simulink model "lab1_1"  (R2020b)
settings: Solver=VariableStepAuto  StartTime=0.0  StopTime=50  MaxStep=0.01  RelTol=1e-3
InitFcn:
  | lambda = 5;
  | theta = 5;
settings Model: Creator=Eeer12  LastModifiedBy=Eugene

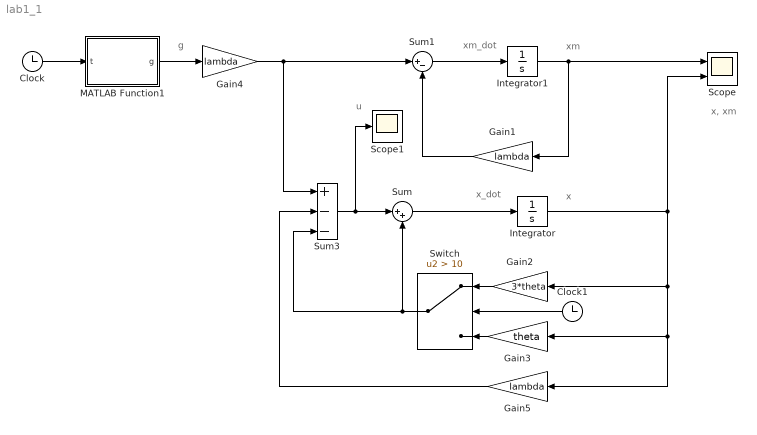
== system lab1_1 ==
  note: x, xm
  note: g
  note: x_dot
  note: x
  note: xm_dot
  note: xm
  note: u
  Clock : Clock
  Clock1 : Clock
  Gain1 : Gain  Gain=lambda
  Gain2 : Gain  Gain=3*theta
  Gain3 : Gain  Gain=theta
  Gain4 : Gain  Gain=lambda
  Gain5 : Gain  Gain=lambda
  Integrator : Integrator
  Integrator1 : Integrator
  MATLAB Function1 : MATLAB Function  TreatAsAtomicUnit=on
  Scope : Scope  NumInputPorts=2
  Scope1 : Scope
  Sum : Sum  Inputs=|++
  Sum1 : Sum  Inputs=|+-
  Sum3 : Sum  Inputs=+--
  Switch : Switch  Criteria=u2 > Threshold  Threshold=10
  wires:
  Integrator/1 -> Scope/2, Gain2/1, Gain3/1, Gain5/1
  Sum/1 -> Integrator/1
  Gain1/1 -> Sum1/2
  Sum1/1 -> Integrator1/1
  Clock1/1 -> Switch/2
  Gain3/1 -> Switch/3
  Clock/1 -> MATLAB Function1/1(t)
  Integrator1/1 -> Scope/1, Gain1/1
  Gain2/1 -> Switch/1
  Switch/1 -> Sum3/3, Sum/2
  Sum3/1 -> Sum/1, Scope1/1
  MATLAB Function1/1(g) -> Gain4/1
  Gain4/1 -> Sum1/1, Sum3/1
  Gain5/1 -> Sum3/2

== matlab function lab1_1/MATLAB Function1 ==
  data: t input; g output
function g = fcn(t)

g = 2*sin(5*t);
